simulink model "hgo_diff"  (R2024b)
settings: Solver=FixedStepAuto  StartTime=0.0  StopTime=15  FixedStep=1e-5  RelTol=1e-3
libraries: simulink x1
settings Model: Creator=user  LastModifiedBy=user

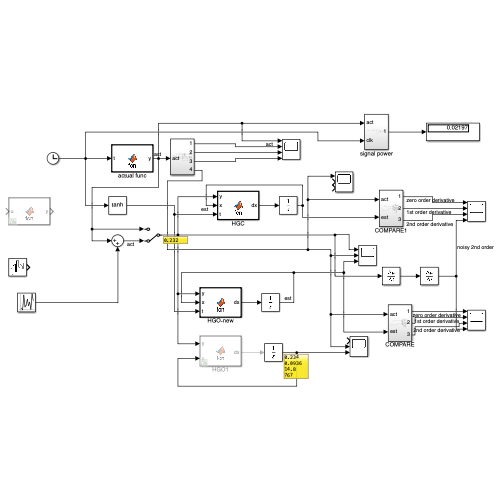
[thumbnail: Simulink's stored preview of the top-level diagram]
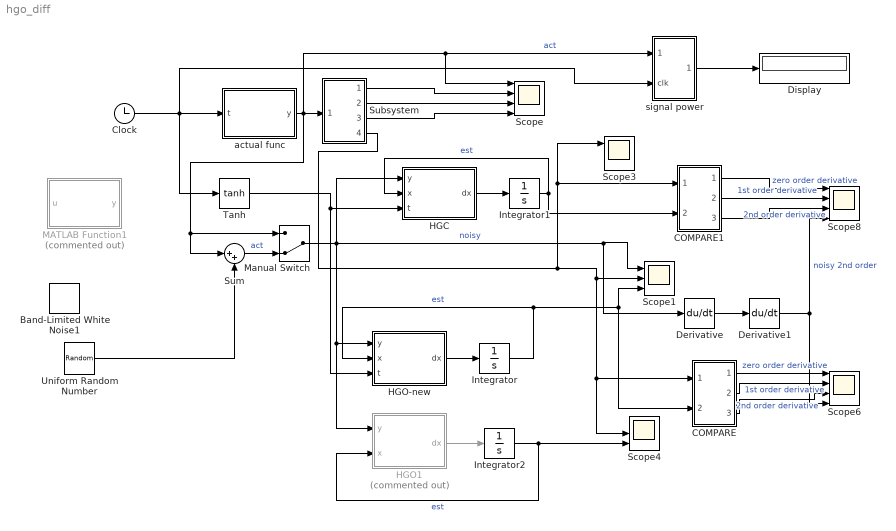
== system hgo_diff ==
  Band-Limited White Noise1 : simulink/Sources/Band-Limited White Noise  Cov=1e-8  Ts=0.001  seed=[23341]
  COMPARE : Subsystem
  COMPARE1 : Subsystem
  Clock : Clock
  Derivative : Derivative
  Derivative1 : Derivative
  Display : Display
  HGC : MATLAB Function  TreatAsAtomicUnit=on
  HGO-new : MATLAB Function  TreatAsAtomicUnit=on
  HGO1 : MATLAB Function  Commented=on  TreatAsAtomicUnit=on
  Integrator : Integrator
  Integrator1 : Integrator
  Integrator2 : Integrator
  MATLAB Function1 : MATLAB Function  Commented=on  TreatAsAtomicUnit=on
  Manual Switch : ManualSwitch  CurrentSetting=0
  Scope : Scope  NumInputPorts=4
  Scope1 : Scope  NumInputPorts=3
  Scope3 : Scope  NumInputPorts=3
  Scope4 : Scope  NumInputPorts=3
  Scope6 : Scope  NumInputPorts=4
  Scope8 : Scope  NumInputPorts=4
  Subsystem : Subsystem
  Sum : Sum  Inputs=|++
  Tanh : Trigonometry  Operator=tanh
  Uniform Random Number : UniformRandomNumber  Minimum=-1e-3  Maximum=1e-3  SampleTime=1e-3
  actual func : MATLAB Function  TreatAsAtomicUnit=on
  signal power : Subsystem
  wires:
  actual func/1(y) -> Manual Switch/1, Sum/1, Subsystem/1(act), signal power/1(act), Scope/1  "act"
  HGO-new/1(dx) -> Integrator/1
  Integrator/1 -> Scope1/3, COMPARE/2(est), HGO-new/2(x)  "est"
  HGC/1(dx) -> Integrator1/1
  Integrator1/1 -> COMPARE1/2(est), HGC/2(x)  "est"
  Sum/1 -> Manual Switch/2  "act"
  Manual Switch/1 -> Scope1/1, Derivative/1, HGC/1(y), HGO-new/1(y), HGO1/1(y)  "noisy"
  HGO1/1(dx) -> Integrator2/1
  Integrator2/1 -> Scope4/3, HGO1/2(x)  "est"
  Clock/1 -> actual func/1(t), signal power/2(clk), Tanh/1
  COMPARE/1(Out1) -> Scope6/1  "zero order derivative"
  COMPARE/2(Out2) -> Scope6/2  "1st order derivative"
  COMPARE/3(Out3) -> Scope6/3  "2nd order derivative"
  Subsystem/4(Out4) -> Scope1/2, COMPARE/1(act), Scope4/2, COMPARE1/1(act), Scope3/1
  Subsystem/1(Out1) -> Scope/2
  Subsystem/2(Out2) -> Scope/3
  Subsystem/3(Out3) -> Scope/4
  COMPARE1/1(Out1) -> Scope8/1  "zero order derivative"
  COMPARE1/2(Out2) -> Scope8/2  "1st order derivative"
  COMPARE1/3(Out3) -> Scope8/3  "2nd order derivative"
  Derivative/1 -> Derivative1/1
  Derivative1/1 -> Scope8/4, Scope6/4  "noisy 2nd order"
  Tanh/1 -> HGO-new/3(t), HGC/3(t)
  Uniform Random Number/1 -> Sum/2
  signal power/1(Out1) -> Display/1

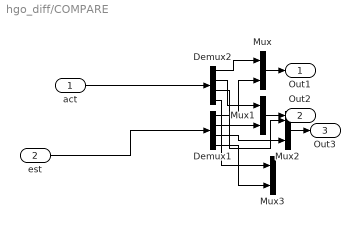
== system hgo_diff/COMPARE ==
  act : Inport
  est : Inport  Port=2
  Demux1 : Demux
  Demux2 : Demux
  Mux{,1..3} (4 alike) : Mux  Inputs=2
  Out1 : Outport
  Out2 : Outport  Port=2
  Out3 : Outport  Port=3
  wires:
  est/1 -> Demux1/1
  Demux1/3 -> Mux2/2
  act/1 -> Demux2/1
  Demux2/1 -> Mux/1
  Mux/1 -> Out1/1
  Demux1/2 -> Mux1/2
  Demux1/1 -> Mux/2
  Demux2/2 -> Mux1/1
  Mux2/1 -> Out3/1
  Demux2/3 -> Mux2/1
  Demux2/4 -> Mux3/1
  Mux1/1 -> Out2/1
  Demux1/4 -> Mux3/2

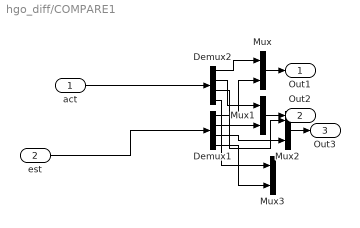
== system hgo_diff/COMPARE1 ==
  act : Inport
  est : Inport  Port=2
  Demux1 : Demux
  Demux2 : Demux
  Mux{,1..3} (4 alike) : Mux  Inputs=2
  Out1 : Outport
  Out2 : Outport  Port=2
  Out3 : Outport  Port=3
  wires:
  Demux1/4 -> Mux3/2
  Mux1/1 -> Out2/1
  Demux2/4 -> Mux3/1
  Demux2/3 -> Mux2/1
  Mux2/1 -> Out3/1
  Demux2/2 -> Mux1/1
  Demux1/1 -> Mux/2
  Demux1/2 -> Mux1/2
  Mux/1 -> Out1/1
  Demux2/1 -> Mux/1
  act/1 -> Demux2/1
  Demux1/3 -> Mux2/2
  est/1 -> Demux1/1

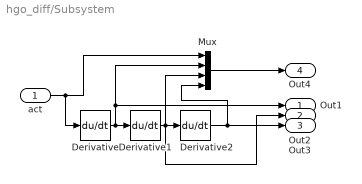
== system hgo_diff/Subsystem ==
  act : Inport
  Derivative : Derivative
  Derivative1 : Derivative
  Derivative2 : Derivative
  Mux : Mux
  Out1 : Outport
  Out2 : Outport  Port=2
  Out3 : Outport  Port=3
  Out4 : Outport  Port=4
  wires:
  Derivative/1 -> Out1/1, Mux/2, Derivative1/1
  Derivative1/1 -> Out2/1, Mux/3, Derivative2/1
  act/1 -> Derivative/1, Mux/1
  Mux/1 -> Out4/1
  Derivative2/1 -> Out3/1, Mux/4

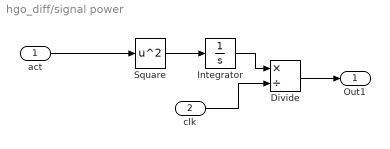
== system hgo_diff/signal power ==
  act : Inport
  clk : Inport  Port=2
  Divide : Product  Inputs=*/
  Integrator : Integrator
  Square : Math  Operator=square
  Out1 : Outport
  wires:
  Square/1 -> Integrator/1
  act/1 -> Square/1
  Integrator/1 -> Divide/1
  clk/1 -> Divide/2
  Divide/1 -> Out1/1

== matlab function hgo_diff/HGC ==
  data: y input; dx output; x input; t input
function dx = fcn(y, x, t)
    % Controllable Canonical Form for n = 4
    % Implements the given equation:
    %   dx_i = x_{i+1},   for 1 ≤ i ≤ n-1
    %   dx_n = -(mu*t)^n * (x_1 - y) - sum( C(n, i) * (mu*t)^i * x_{n-i+1} )

    % Order of observer
    n = 4;
    mu = 90; % hgo gain 
    t = t/5; % scaling factor compromise between peak and accuracy
    %a = 1; 
    %t = 1;

    % Ci = nchoosek(n, i)
    C = [4, 6, 4, 1];

    % Initialize derivative vector
    dx = zeros(n, 1);

    % First three equations: dx_i = x_{i+1}
    dx(1) = x(2);
    dx(2) = x(3);
    dx(3) = x(4);

    % Compute dx_4 using the given formula
    dx(4) = - (mu*t)^4 * (x(1) - y) - (C(1)*(mu*t)^1*x(4)) ... 
            - (C(2)*(mu*t)^2* x(3)) - (C(3)*(mu*t)^3*x(2));
end

== matlab function hgo_diff/actual func ==
  data: t input; y output
function y = fcn(t)
y = -(1 + exp(-2*t)) * sin(2*t)/(5 + cos(t));
%y = -cos(t)/(2+sin(3*t));
% y = sin(t) + cos(5*t);
% dy = cos(t) - 5*sin(5*t);
% d2y = -sin(t) - 25*cos(5*t);
% d3y = -cos(t) + 125*sin(5*t);
% d4y = sin(t) + 625*cos(5*t);

% yt = [y; dy; d2y; d3y];

== matlab function hgo_diff/HGO-new ==
  data: y input; dx output; x input; t input
function dx = fcn(y, x, t)
    % Parameters
    n = 4;                % Order of the observer
    epsilon = 1/200;      % Small gain parameter
    tr = t/10; 
    % Binomial coefficients (for n = 4)
    % ki = nchoosek(n, i)
    k = [4, 6, 4, 1]; 

    e = 1e-5;
    % Initialize output derivative
    dx = zeros(n, 1);
    
    % High-Gain Observer Equations
    dx(1) = x(2) + (k(1)*(tr+e)^1 / epsilon^1) * (y - x(1));
    dx(2) = x(3) + (k(2)*(tr+e)^2 / epsilon^2) * (y - x(1));
    dx(3) = x(4) + (k(3)*(tr+e)^3 / epsilon^3) * (y - x(1));
    dx(4) = (k(4)*(tr+e)^4 / epsilon^4) * (y - x(1));
end

== matlab function hgo_diff/HGO1 ==
  data: y input; dx output; x input
function dx = fcn(y, x)
    % Parameters
    n = 4;                % Order of the observer
    epsilon = 1/200;      % Small gain parameter
    % tr = 1 ; 
    % Binomial coefficients (for n = 4)
    % ki = nchoosek(n, i)
    k = [4, 6, 4, 1]; 

    % Initialize output derivative
    dx = zeros(n, 1);
    
    % High-Gain Observer Equations
    dx(1) = x(2) + (k(1) / epsilon^1) * (y - x(1));
    dx(2) = x(3) + (k(2) / epsilon^2) * (y - x(1));
    dx(3) = x(4) + (k(3) / epsilon^3) * (y - x(1));
    dx(4) = (k(4) / epsilon^4) * (y - x(1));
end

== matlab function hgo_diff/MATLAB Function1 ==
  data: u input; y output
function y = fcn(u)

y = u;
